simulink model "gm_uz_pmsm_model_6LUT_pd"  (R2023b)
settings: Solver=FixedStepAuto  StartTime=0.0  StopTime=0.05  RelTol=1e-3
PreLoadFcn:
  | uz_pmsm_model_init_parameter
PostLoadFcn:
  | % Import the data from Excel for a lookup table
  | FluxMapData = readtable('C:\Users\Philipp\ultrazohm\ultrazohm_sw\ip_cores\uz_pmsm_model\FluxMapData_2023-05-26_13-07-57.csv');
  | % Row indices for lookup table
  | d_current_in_d_axis = FluxMapData(8:27,1:end);
  | % Column indices for lookup table
  | q_current_in_d_axis = FluxMapData(29:48,1:end);
  | % Output values for lookup table
  | d_Flux_d_axis = FluxMapData(50:69,1:end);
undefined symbols (not defined in the file or in its folder): ad1, ad2, ad3, ad4, ad5, ad6, aq1, aq2, aq3, aq4, aq5, aq6, d_current_d_Flux, d_current_q_Flux, entkopplung_dynamic, entkopplung_linear, entkopplung_static, Fid1_Giq1, Fid2_Giq2, Flux_d, Flux_q, friction_coefficient, inertia, Ki_Bo_d, Ki_Bo_q, Kp_Bo_d, Kp_Bo_q, L_d, L_q, Ldq, parameter_nachfuerung, polepair, praediktion_entkopplung_nonlinear, psi_pm, q_current_d_Flux, q_current_q_Flux, R_1, simulate_mechanical, simulate_nonlinear_modell, simulate_open_loop, static_friction_torque, tau_sum, ts_regler
libraries: hdlmdlgenlib x21, slpidlib x2
(part 3 of 3)

== system gm_uz_pmsm_model_6LUT_pd/uz_pmsm_model/Product142 ==
  In1 : Inport
  In2 : Inport  Port=2
  Product142 : Product  Inputs=**  OutDataTypeStr=single  SampleTime=1e-08
  Product142_pd1 : Delay  DelayLength=6
  Out1 : Outport
  wires:
  In1/1 -> Product142/1
  In2/1 -> Product142/2
  Product142/1 -> Product142_pd1/1
  Product142_pd1/1 -> Out1/1

== system gm_uz_pmsm_model_6LUT_pd/uz_pmsm_model/Product15 ==
  In1 : Inport
  In2 : Inport  Port=2
  Product15 : Product  Inputs=**  OutDataTypeStr=single  SampleTime=1e-08
  Product15_pd1 : Delay  DelayLength=6
  Out1 : Outport
  wires:
  In1/1 -> Product15/1
  In2/1 -> Product15/2
  Product15/1 -> Product15_pd1/1
  Product15_pd1/1 -> Out1/1

== system gm_uz_pmsm_model_6LUT_pd/uz_pmsm_model/Product151 ==
  In1 : Inport
  In2 : Inport  Port=2
  Product151 : Product  Inputs=**  OutDataTypeStr=single  SampleTime=1e-08
  Product151_pd1 : Delay  DelayLength=6
  Out1 : Outport
  wires:
  In1/1 -> Product151/1
  In2/1 -> Product151/2
  Product151/1 -> Product151_pd1/1
  Product151_pd1/1 -> Out1/1

== system gm_uz_pmsm_model_6LUT_pd/uz_pmsm_model/Product16 ==
  In1 : Inport
  In2 : Inport  Port=2
  Product16 : Product  Inputs=**  OutDataTypeStr=single  SampleTime=1e-08
  Product16_pd1 : Delay  DelayLength=6
  Out1 : Outport
  wires:
  In1/1 -> Product16/1
  In2/1 -> Product16/2
  Product16/1 -> Product16_pd1/1
  Product16_pd1/1 -> Out1/1

== system gm_uz_pmsm_model_6LUT_pd/uz_pmsm_model/Product17 ==
  In1 : Inport
  In2 : Inport  Port=2
  Product17 : Product  Inputs=**  OutDataTypeStr=single  SampleTime=1e-08
  Product17_pd1 : Delay  DelayLength=6
  Out1 : Outport
  wires:
  In1/1 -> Product17/1
  In2/1 -> Product17/2
  Product17/1 -> Product17_pd1/1
  Product17_pd1/1 -> Out1/1

== system gm_uz_pmsm_model_6LUT_pd/uz_pmsm_model/Product18 ==
  In1 : Inport
  In2 : Inport  Port=2
  Product18 : Product  Inputs=**  OutDataTypeStr=single  SampleTime=1e-08
  Product18_pd1 : Delay  DelayLength=6
  Out1 : Outport
  wires:
  In1/1 -> Product18/1
  In2/1 -> Product18/2
  Product18/1 -> Product18_pd1/1
  Product18_pd1/1 -> Out1/1

== system gm_uz_pmsm_model_6LUT_pd/uz_pmsm_model/Product19 ==
  In1 : Inport
  In2 : Inport  Port=2
  Product19 : Product  Inputs=**  OutDataTypeStr=single  SampleTime=1e-08
  Product19_pd1 : Delay  DelayLength=6
  Out1 : Outport
  wires:
  In1/1 -> Product19/1
  In2/1 -> Product19/2
  Product19/1 -> Product19_pd1/1
  Product19_pd1/1 -> Out1/1

== system gm_uz_pmsm_model_6LUT_pd/uz_pmsm_model/Product2 ==
  In1 : Inport
  In2 : Inport  Port=2
  Product2 : Product  Inputs=**  OutDataTypeStr=single  SampleTime=1e-08
  Product2_pd1 : Delay  DelayLength=6
  Out1 : Outport
  wires:
  In1/1 -> Product2/1
  In2/1 -> Product2/2
  Product2/1 -> Product2_pd1/1
  Product2_pd1/1 -> Out1/1

== system gm_uz_pmsm_model_6LUT_pd/uz_pmsm_model/Product20 ==
  In1 : Inport
  In2 : Inport  Port=2
  Product20 : Product  Inputs=**  OutDataTypeStr=single  SampleTime=1e-08
  Product20_pd1 : Delay  DelayLength=6
  Out1 : Outport
  wires:
  In1/1 -> Product20/1
  In2/1 -> Product20/2
  Product20/1 -> Product20_pd1/1
  Product20_pd1/1 -> Out1/1

== system gm_uz_pmsm_model_6LUT_pd/uz_pmsm_model/Product201 ==
  In1 : Inport
  In2 : Inport  Port=2
  Product201 : Product  Inputs=**  OutDataTypeStr=single  SampleTime=1e-08
  Product201_pd1 : Delay  DelayLength=6
  Out1 : Outport
  wires:
  In1/1 -> Product201/1
  In2/1 -> Product201/2
  Product201/1 -> Product201_pd1/1
  Product201_pd1/1 -> Out1/1

== system gm_uz_pmsm_model_6LUT_pd/uz_pmsm_model/Product202 ==
  In1 : Inport
  In2 : Inport  Port=2
  Product202 : Product  Inputs=**  OutDataTypeStr=single  SampleTime=1e-08
  Product202_pd1 : Delay  DelayLength=6
  Out1 : Outport
  wires:
  In1/1 -> Product202/1
  In2/1 -> Product202/2
  Product202/1 -> Product202_pd1/1
  Product202_pd1/1 -> Out1/1

== system gm_uz_pmsm_model_6LUT_pd/uz_pmsm_model/Product203 ==
  In1 : Inport
  In2 : Inport  Port=2
  Product203 : Product  Inputs=**  OutDataTypeStr=single  SampleTime=1e-08
  Product203_pd1 : Delay  DelayLength=6
  Out1 : Outport
  wires:
  In1/1 -> Product203/1
  In2/1 -> Product203/2
  Product203/1 -> Product203_pd1/1
  Product203_pd1/1 -> Out1/1

== system gm_uz_pmsm_model_6LUT_pd/uz_pmsm_model/Product204 ==
  In1 : Inport
  In2 : Inport  Port=2
  Product204 : Product  Inputs=**  OutDataTypeStr=single  SampleTime=1e-08
  Product204_pd1 : Delay  DelayLength=6
  Out1 : Outport
  wires:
  In1/1 -> Product204/1
  In2/1 -> Product204/2
  Product204/1 -> Product204_pd1/1
  Product204_pd1/1 -> Out1/1

== system gm_uz_pmsm_model_6LUT_pd/uz_pmsm_model/Product205 ==
  In1 : Inport
  In2 : Inport  Port=2
  Product205 : Product  Inputs=**  OutDataTypeStr=single  SampleTime=1e-08
  Product205_pd1 : Delay  DelayLength=6
  Out1 : Outport
  wires:
  In1/1 -> Product205/1
  In2/1 -> Product205/2
  Product205/1 -> Product205_pd1/1
  Product205_pd1/1 -> Out1/1

== system gm_uz_pmsm_model_6LUT_pd/uz_pmsm_model/Product206 ==
  In1 : Inport
  In2 : Inport  Port=2
  Product206 : Product  Inputs=**  OutDataTypeStr=single  SampleTime=1e-08
  Product206_pd1 : Delay  DelayLength=6
  Out1 : Outport
  wires:
  In1/1 -> Product206/1
  In2/1 -> Product206/2
  Product206/1 -> Product206_pd1/1
  Product206_pd1/1 -> Out1/1

== system gm_uz_pmsm_model_6LUT_pd/uz_pmsm_model/Product207 ==
  In1 : Inport
  In2 : Inport  Port=2
  Product207 : Product  Inputs=**  OutDataTypeStr=single  SampleTime=1e-08
  Product207_pd1 : Delay  DelayLength=6
  Out1 : Outport
  wires:
  In1/1 -> Product207/1
  In2/1 -> Product207/2
  Product207/1 -> Product207_pd1/1
  Product207_pd1/1 -> Out1/1

== system gm_uz_pmsm_model_6LUT_pd/uz_pmsm_model/Product21 ==
  In1 : Inport
  In2 : Inport  Port=2
  Product21 : Product  Inputs=**  OutDataTypeStr=single  SampleTime=1e-08
  Product21_pd1 : Delay  DelayLength=6
  Out1 : Outport
  wires:
  In1/1 -> Product21/1
  In2/1 -> Product21/2
  Product21/1 -> Product21_pd1/1
  Product21_pd1/1 -> Out1/1

== system gm_uz_pmsm_model_6LUT_pd/uz_pmsm_model/Product22 ==
  In1 : Inport
  In2 : Inport  Port=2
  Product22 : Product  Inputs=**  OutDataTypeStr=single  SampleTime=1e-08
  Product22_pd1 : Delay  DelayLength=6
  Out1 : Outport
  wires:
  In1/1 -> Product22/1
  In2/1 -> Product22/2
  Product22/1 -> Product22_pd1/1
  Product22_pd1/1 -> Out1/1

== system gm_uz_pmsm_model_6LUT_pd/uz_pmsm_model/Product23 ==
  In1 : Inport
  In2 : Inport  Port=2
  Product23 : Product  Inputs=**  OutDataTypeStr=single  SampleTime=1e-08
  Product23_pd1 : Delay  DelayLength=6
  Out1 : Outport
  wires:
  In1/1 -> Product23/1
  In2/1 -> Product23/2
  Product23/1 -> Product23_pd1/1
  Product23_pd1/1 -> Out1/1

== system gm_uz_pmsm_model_6LUT_pd/uz_pmsm_model/Product24 ==
  In1 : Inport
  In2 : Inport  Port=2
  Product24 : Product  Inputs=**  OutDataTypeStr=single  SampleTime=1e-08
  Product24_pd1 : Delay  DelayLength=6
  Out1 : Outport
  wires:
  In1/1 -> Product24/1
  In2/1 -> Product24/2
  Product24/1 -> Product24_pd1/1
  Product24_pd1/1 -> Out1/1

== system gm_uz_pmsm_model_6LUT_pd/uz_pmsm_model/Product25 ==
  In1 : Inport
  In2 : Inport  Port=2
  Product25 : Product  Inputs=**  OutDataTypeStr=single  SampleTime=1e-08
  Product25_pd1 : Delay  DelayLength=6
  Out1 : Outport
  wires:
  In1/1 -> Product25/1
  In2/1 -> Product25/2
  Product25/1 -> Product25_pd1/1
  Product25_pd1/1 -> Out1/1

== system gm_uz_pmsm_model_6LUT_pd/uz_pmsm_model/Product3 ==
  In1 : Inport
  In2 : Inport  Port=2
  Product3 : Product  Inputs=**  OutDataTypeStr=single  SampleTime=1e-08
  Product3_pd1 : Delay  DelayLength=6
  Out1 : Outport
  wires:
  In1/1 -> Product3/1
  In2/1 -> Product3/2
  Product3/1 -> Product3_pd1/1
  Product3_pd1/1 -> Out1/1

== system gm_uz_pmsm_model_6LUT_pd/uz_pmsm_model/Product31 ==
  In1 : Inport
  In2 : Inport  Port=2
  Product31 : Product  Inputs=**  OutDataTypeStr=single  SampleTime=1e-08
  Product31_pd1 : Delay  DelayLength=6
  Out1 : Outport
  wires:
  In1/1 -> Product31/1
  In2/1 -> Product31/2
  Product31/1 -> Product31_pd1/1
  Product31_pd1/1 -> Out1/1

== system gm_uz_pmsm_model_6LUT_pd/uz_pmsm_model/Product32 ==
  In1 : Inport
  In2 : Inport  Port=2
  Product32 : Product  Inputs=**  OutDataTypeStr=single  SampleTime=1e-08
  Product32_pd1 : Delay  DelayLength=6
  Out1 : Outport
  wires:
  In1/1 -> Product32/1
  In2/1 -> Product32/2
  Product32/1 -> Product32_pd1/1
  Product32_pd1/1 -> Out1/1

== system gm_uz_pmsm_model_6LUT_pd/uz_pmsm_model/Product33 ==
  In1 : Inport
  In2 : Inport  Port=2
  Product33 : Product  Inputs=**  OutDataTypeStr=single  SampleTime=1e-08
  Product33_pd1 : Delay  DelayLength=6
  Out1 : Outport
  wires:
  In1/1 -> Product33/1
  In2/1 -> Product33/2
  Product33/1 -> Product33_pd1/1
  Product33_pd1/1 -> Out1/1

== system gm_uz_pmsm_model_6LUT_pd/uz_pmsm_model/Product34 ==
  In1 : Inport
  In2 : Inport  Port=2
  Product34 : Product  Inputs=**  OutDataTypeStr=single  SampleTime=1e-08
  Product34_pd1 : Delay  DelayLength=6
  Out1 : Outport
  wires:
  In1/1 -> Product34/1
  In2/1 -> Product34/2
  Product34/1 -> Product34_pd1/1
  Product34_pd1/1 -> Out1/1

== system gm_uz_pmsm_model_6LUT_pd/uz_pmsm_model/Product35 ==
  In1 : Inport
  In2 : Inport  Port=2
  Product35 : Product  Inputs=**  OutDataTypeStr=single  SampleTime=1e-08
  Product35_pd1 : Delay  DelayLength=6
  Out1 : Outport
  wires:
  In1/1 -> Product35/1
  In2/1 -> Product35/2
  Product35/1 -> Product35_pd1/1
  Product35_pd1/1 -> Out1/1

== system gm_uz_pmsm_model_6LUT_pd/uz_pmsm_model/Product4 ==
  In1 : Inport
  In2 : Inport  Port=2
  Product4 : Product  Inputs=**  OutDataTypeStr=single  SampleTime=1e-08
  Product4_pd1 : Delay  DelayLength=6
  Out1 : Outport
  wires:
  In1/1 -> Product4/1
  In2/1 -> Product4/2
  Product4/1 -> Product4_pd1/1
  Product4_pd1/1 -> Out1/1

== system gm_uz_pmsm_model_6LUT_pd/uz_pmsm_model/Product41 ==
  In1 : Inport
  In2 : Inport  Port=2
  Product41 : Product  Inputs=**  OutDataTypeStr=single  SampleTime=1e-08
  Product41_pd1 : Delay  DelayLength=6
  Out1 : Outport
  wires:
  In1/1 -> Product41/1
  In2/1 -> Product41/2
  Product41/1 -> Product41_pd1/1
  Product41_pd1/1 -> Out1/1

== system gm_uz_pmsm_model_6LUT_pd/uz_pmsm_model/Product42 ==
  In1 : Inport
  In2 : Inport  Port=2
  Product42 : Product  Inputs=**  OutDataTypeStr=single  SampleTime=1e-08
  Product42_pd1 : Delay  DelayLength=6
  Out1 : Outport
  wires:
  In1/1 -> Product42/1
  In2/1 -> Product42/2
  Product42/1 -> Product42_pd1/1
  Product42_pd1/1 -> Out1/1

== system gm_uz_pmsm_model_6LUT_pd/uz_pmsm_model/Product43 ==
  In1 : Inport
  In2 : Inport  Port=2
  Product43 : Product  Inputs=**  OutDataTypeStr=single  SampleTime=1e-08
  Product43_pd1 : Delay  DelayLength=6
  Out1 : Outport
  wires:
  In1/1 -> Product43/1
  In2/1 -> Product43/2
  Product43/1 -> Product43_pd1/1
  Product43_pd1/1 -> Out1/1

== system gm_uz_pmsm_model_6LUT_pd/uz_pmsm_model/Product5 ==
  In1 : Inport
  In2 : Inport  Port=2
  Product5 : Product  Inputs=**  OutDataTypeStr=single  SampleTime=1e-08
  Product5_pd1 : Delay  DelayLength=6
  Out1 : Outport
  wires:
  In1/1 -> Product5/1
  In2/1 -> Product5/2
  Product5/1 -> Product5_pd1/1
  Product5_pd1/1 -> Out1/1

== system gm_uz_pmsm_model_6LUT_pd/uz_pmsm_model/Product51 ==
  In1 : Inport
  In2 : Inport  Port=2
  Product51 : Product  Inputs=**  OutDataTypeStr=single  SampleTime=1e-08
  Product51_pd1 : Delay  DelayLength=6
  Out1 : Outport
  wires:
  In1/1 -> Product51/1
  In2/1 -> Product51/2
  Product51/1 -> Product51_pd1/1
  Product51_pd1/1 -> Out1/1

== system gm_uz_pmsm_model_6LUT_pd/uz_pmsm_model/Product52 ==
  In1 : Inport
  In2 : Inport  Port=2
  Product52 : Product  Inputs=**  OutDataTypeStr=single  SampleTime=1e-08
  Product52_pd1 : Delay  DelayLength=6
  Out1 : Outport
  wires:
  In1/1 -> Product52/1
  In2/1 -> Product52/2
  Product52/1 -> Product52_pd1/1
  Product52_pd1/1 -> Out1/1

== system gm_uz_pmsm_model_6LUT_pd/uz_pmsm_model/Product6 ==
  In1 : Inport
  In2 : Inport  Port=2
  Product6 : Product  Inputs=**  OutDataTypeStr=single  SampleTime=1e-08
  Product6_pd1 : Delay  DelayLength=6
  Out1 : Outport
  wires:
  In1/1 -> Product6/1
  In2/1 -> Product6/2
  Product6/1 -> Product6_pd1/1
  Product6_pd1/1 -> Out1/1

== system gm_uz_pmsm_model_6LUT_pd/uz_pmsm_model/Product61 ==
  In1 : Inport
  In2 : Inport  Port=2
  Product61 : Product  Inputs=**  OutDataTypeStr=single  SampleTime=1e-08
  Product61_pd1 : Delay  DelayLength=6
  Out1 : Outport
  wires:
  In1/1 -> Product61/1
  In2/1 -> Product61/2
  Product61/1 -> Product61_pd1/1
  Product61_pd1/1 -> Out1/1

== system gm_uz_pmsm_model_6LUT_pd/uz_pmsm_model/Product7 ==
  In1 : Inport
  In2 : Inport  Port=2
  Product7 : Product  Inputs=**  OutDataTypeStr=single  SampleTime=1e-08
  Product7_pd1 : Delay  DelayLength=6
  Out1 : Outport
  wires:
  In1/1 -> Product7/1
  In2/1 -> Product7/2
  Product7/1 -> Product7_pd1/1
  Product7_pd1/1 -> Out1/1

== system gm_uz_pmsm_model_6LUT_pd/uz_pmsm_model/Product71 ==
  In1 : Inport
  In2 : Inport  Port=2
  Product71 : Product  Inputs=**  OutDataTypeStr=single  SampleTime=1e-08
  Product71_pd1 : Delay  DelayLength=6
  Out1 : Outport
  wires:
  In1/1 -> Product71/1
  In2/1 -> Product71/2
  Product71/1 -> Product71_pd1/1
  Product71_pd1/1 -> Out1/1

== system gm_uz_pmsm_model_6LUT_pd/uz_pmsm_model/Product8 ==
  In1 : Inport
  In2 : Inport  Port=2
  Product8 : Product  Inputs=**  OutDataTypeStr=single  SampleTime=1e-08
  Product8_pd1 : Delay  DelayLength=6
  Out1 : Outport
  wires:
  In1/1 -> Product8/1
  In2/1 -> Product8/2
  Product8/1 -> Product8_pd1/1
  Product8_pd1/1 -> Out1/1

== system gm_uz_pmsm_model_6LUT_pd/uz_pmsm_model/Product9 ==
  In1 : Inport
  In2 : Inport  Port=2
  Product9 : Product  Inputs=**  OutDataTypeStr=single  SampleTime=1e-08
  Product9_pd1 : Delay  DelayLength=6
  Out1 : Outport
  wires:
  In1/1 -> Product9/1
  In2/1 -> Product9/2
  Product9/1 -> Product9_pd1/1
  Product9_pd1/1 -> Out1/1

== system gm_uz_pmsm_model_6LUT_pd/uz_pmsm_model/Product91 ==
  In1 : Inport
  In2 : Inport  Port=2
  Product91 : Product  Inputs=**  OutDataTypeStr=single  SampleTime=1e-08
  Product91_pd1 : Delay  DelayLength=6
  Out1 : Outport
  wires:
  In1/1 -> Product91/1
  In2/1 -> Product91/2
  Product91/1 -> Product91_pd1/1
  Product91_pd1/1 -> Out1/1

== system gm_uz_pmsm_model_6LUT_pd/uz_pmsm_model/Product92 ==
  In1 : Inport
  In2 : Inport  Port=2
  Product92 : Product  Inputs=**  OutDataTypeStr=single  SampleTime=1e-08
  Product92_pd1 : Delay  DelayLength=6
  Out1 : Outport
  wires:
  In1/1 -> Product92/1
  In2/1 -> Product92/2
  Product92/1 -> Product92_pd1/1
  Product92_pd1/1 -> Out1/1

== system gm_uz_pmsm_model_6LUT_pd/uz_pmsm_model/Reciprocal1_recip ==
  In1 : Inport
  Reciprocal1_recip : Math  Operator=reciprocal  SampleTime=1e-08
  Reciprocal1_recip_pd1 : Delay  DelayLength=16
  Out1 : Outport
  wires:
  In1/1 -> Reciprocal1_recip/1
  Reciprocal1_recip/1 -> Reciprocal1_recip_pd1/1
  Reciprocal1_recip_pd1/1 -> Out1/1

== system gm_uz_pmsm_model_6LUT_pd/uz_pmsm_model/Reciprocal1_recip1 ==
  In1 : Inport
  Reciprocal1_recip1 : Math  Operator=reciprocal  SampleTime=1e-08
  Reciprocal1_recip1_pd1 : Delay  DelayLength=16
  Out1 : Outport
  wires:
  In1/1 -> Reciprocal1_recip1/1
  Reciprocal1_recip1/1 -> Reciprocal1_recip1_pd1/1
  Reciprocal1_recip1_pd1/1 -> Out1/1

== system gm_uz_pmsm_model_6LUT_pd/uz_pmsm_model/Reciprocal_recip ==
  In1 : Inport
  Reciprocal_recip : Math  Operator=reciprocal  SampleTime=1e-08
  Reciprocal_recip_pd1 : Delay  DelayLength=16
  Out1 : Outport
  wires:
  In1/1 -> Reciprocal_recip/1
  Reciprocal_recip/1 -> Reciprocal_recip_pd1/1
  Reciprocal_recip_pd1/1 -> Out1/1

== system gm_uz_pmsm_model_6LUT_pd/uz_pmsm_model/Reciprocal_recip1 ==
  In1 : Inport
  Reciprocal_recip1 : Math  Operator=reciprocal  SampleTime=1e-08
  Reciprocal_recip1_pd1 : Delay  DelayLength=16
  Out1 : Outport
  wires:
  In1/1 -> Reciprocal_recip1/1
  Reciprocal_recip1/1 -> Reciprocal_recip1_pd1/1
  Reciprocal_recip1_pd1/1 -> Out1/1

== system gm_uz_pmsm_model_6LUT_pd/uz_pmsm_model/Sign1 ==
  In1 : Inport
  Sign1 : Signum  SampleTime=1e-08
  Out1 : Outport
  wires:
  In1/1 -> Sign1/1
  Sign1/1 -> Out1/1

== system gm_uz_pmsm_model_6LUT_pd/uz_pmsm_model/Sum ==
  In1 : Inport
  In2 : Inport  Port=2
  Sum : Sum  OutDataTypeStr=single  SampleTime=1e-08
  Sum_pd1 : Delay  DelayLength=6
  Out1 : Outport
  wires:
  In1/1 -> Sum/1
  In2/1 -> Sum/2
  Sum/1 -> Sum_pd1/1
  Sum_pd1/1 -> Out1/1

== system gm_uz_pmsm_model_6LUT_pd/uz_pmsm_model/Sum1 ==
  In1 : Inport
  In2 : Inport  Port=2
  Sum1 : Sum  Inputs=+-  OutDataTypeStr=single  SampleTime=1e-08
  Sum1_pd1 : Delay  DelayLength=6
  Out1 : Outport
  wires:
  In1/1 -> Sum1/1
  In2/1 -> Sum1/2
  Sum1/1 -> Sum1_pd1/1
  Sum1_pd1/1 -> Out1/1

== system gm_uz_pmsm_model_6LUT_pd/uz_pmsm_model/Sum10 ==
  In1 : Inport
  In2 : Inport  Port=2
  Sum10 : Sum  Inputs=+-  OutDataTypeStr=single  SampleTime=1e-08
  Sum10_pd1 : Delay  DelayLength=6
  Out1 : Outport
  wires:
  In1/1 -> Sum10/1
  In2/1 -> Sum10/2
  Sum10/1 -> Sum10_pd1/1
  Sum10_pd1/1 -> Out1/1

== system gm_uz_pmsm_model_6LUT_pd/uz_pmsm_model/Sum101 ==
  In1 : Inport
  In2 : Inport  Port=2
  Sum101 : Sum  Inputs=+-  OutDataTypeStr=single  SampleTime=1e-08
  Sum101_pd1 : Delay  DelayLength=6
  Out1 : Outport
  wires:
  In1/1 -> Sum101/1
  In2/1 -> Sum101/2
  Sum101/1 -> Sum101_pd1/1
  Sum101_pd1/1 -> Out1/1

== system gm_uz_pmsm_model_6LUT_pd/uz_pmsm_model/Sum11 ==
  In1 : Inport
  In2 : Inport  Port=2
  Sum11 : Sum  Inputs=+-  OutDataTypeStr=single  SampleTime=1e-08
  Sum11_pd1 : Delay  DelayLength=6
  Out1 : Outport
  wires:
  In1/1 -> Sum11/1
  In2/1 -> Sum11/2
  Sum11/1 -> Sum11_pd1/1
  Sum11_pd1/1 -> Out1/1

== system gm_uz_pmsm_model_6LUT_pd/uz_pmsm_model/Sum12 ==
  In1 : Inport
  In2 : Inport  Port=2
  Sum12 : Sum  OutDataTypeStr=single  SampleTime=1e-08
  Sum12_pd1 : Delay  DelayLength=6
  Out1 : Outport
  wires:
  In1/1 -> Sum12/1
  In2/1 -> Sum12/2
  Sum12/1 -> Sum12_pd1/1
  Sum12_pd1/1 -> Out1/1

== system gm_uz_pmsm_model_6LUT_pd/uz_pmsm_model/Sum13 ==
  In1 : Inport
  In2 : Inport  Port=2
  Sum13 : Sum  OutDataTypeStr=single  SampleTime=1e-08
  Sum13_pd1 : Delay  DelayLength=6
  Out1 : Outport
  wires:
  In1/1 -> Sum13/1
  In2/1 -> Sum13/2
  Sum13/1 -> Sum13_pd1/1
  Sum13_pd1/1 -> Out1/1

== system gm_uz_pmsm_model_6LUT_pd/uz_pmsm_model/Sum14 ==
  In1 : Inport
  In2 : Inport  Port=2
  Sum14 : Sum  Inputs=+-  OutDataTypeStr=single  SampleTime=1e-08
  Sum14_pd1 : Delay  DelayLength=6
  Out1 : Outport
  wires:
  In1/1 -> Sum14/1
  In2/1 -> Sum14/2
  Sum14/1 -> Sum14_pd1/1
  Sum14_pd1/1 -> Out1/1

== system gm_uz_pmsm_model_6LUT_pd/uz_pmsm_model/Sum2 ==
  In1 : Inport
  In2 : Inport  Port=2
  Sum2 : Sum  Inputs=+-  OutDataTypeStr=single  SampleTime=1e-08
  Sum2_pd1 : Delay  DelayLength=6
  Out1 : Outport
  wires:
  In1/1 -> Sum2/1
  In2/1 -> Sum2/2
  Sum2/1 -> Sum2_pd1/1
  Sum2_pd1/1 -> Out1/1

== system gm_uz_pmsm_model_6LUT_pd/uz_pmsm_model/Sum21 ==
  In1 : Inport
  In2 : Inport  Port=2
  Sum21 : Sum  Inputs=+-  OutDataTypeStr=single  SampleTime=1e-08
  Sum21_pd1 : Delay  DelayLength=6
  Out1 : Outport
  wires:
  In1/1 -> Sum21/1
  In2/1 -> Sum21/2
  Sum21/1 -> Sum21_pd1/1
  Sum21_pd1/1 -> Out1/1

== system gm_uz_pmsm_model_6LUT_pd/uz_pmsm_model/Sum22 ==
  In1 : Inport
  In2 : Inport  Port=2
  Sum22 : Sum  Inputs=+-  OutDataTypeStr=single  SampleTime=1e-08
  Sum22_pd1 : Delay  DelayLength=6
  Out1 : Outport
  wires:
  In1/1 -> Sum22/1
  In2/1 -> Sum22/2
  Sum22/1 -> Sum22_pd1/1
  Sum22_pd1/1 -> Out1/1

== system gm_uz_pmsm_model_6LUT_pd/uz_pmsm_model/Sum23 ==
  In1 : Inport
  In2 : Inport  Port=2
  Sum23 : Sum  Inputs=+-  OutDataTypeStr=single  SampleTime=1e-08
  Sum23_pd1 : Delay  DelayLength=6
  Out1 : Outport
  wires:
  In1/1 -> Sum23/1
  In2/1 -> Sum23/2
  Sum23/1 -> Sum23_pd1/1
  Sum23_pd1/1 -> Out1/1

== system gm_uz_pmsm_model_6LUT_pd/uz_pmsm_model/Sum3 ==
  In1 : Inport
  In2 : Inport  Port=2
  Sum3 : Sum  Inputs=+-  OutDataTypeStr=single  SampleTime=1e-08
  Sum3_pd1 : Delay  DelayLength=6
  Out1 : Outport
  wires:
  In1/1 -> Sum3/1
  In2/1 -> Sum3/2
  Sum3/1 -> Sum3_pd1/1
  Sum3_pd1/1 -> Out1/1

== system gm_uz_pmsm_model_6LUT_pd/uz_pmsm_model/Sum31 ==
  In1 : Inport
  In2 : Inport  Port=2
  Sum31 : Sum  Inputs=+-  OutDataTypeStr=single  SampleTime=1e-08
  Sum31_pd1 : Delay  DelayLength=6
  Out1 : Outport
  wires:
  In1/1 -> Sum31/1
  In2/1 -> Sum31/2
  Sum31/1 -> Sum31_pd1/1
  Sum31_pd1/1 -> Out1/1

== system gm_uz_pmsm_model_6LUT_pd/uz_pmsm_model/Sum32 ==
  In1 : Inport
  In2 : Inport  Port=2
  Sum32 : Sum  OutDataTypeStr=single  SampleTime=1e-08
  Sum32_pd1 : Delay  DelayLength=6
  Out1 : Outport
  wires:
  In1/1 -> Sum32/1
  In2/1 -> Sum32/2
  Sum32/1 -> Sum32_pd1/1
  Sum32_pd1/1 -> Out1/1

== system gm_uz_pmsm_model_6LUT_pd/uz_pmsm_model/Sum33 ==
  In1 : Inport
  In2 : Inport  Port=2
  Sum33 : Sum  Inputs=+-  OutDataTypeStr=single  SampleTime=1e-08
  Sum33_pd1 : Delay  DelayLength=6
  Out1 : Outport
  wires:
  In1/1 -> Sum33/1
  In2/1 -> Sum33/2
  Sum33/1 -> Sum33_pd1/1
  Sum33_pd1/1 -> Out1/1

== system gm_uz_pmsm_model_6LUT_pd/uz_pmsm_model/Sum3_stage2 ==
  In1 : Inport
  In2 : Inport  Port=2
  Sum3_stage2 : Sum  OutDataTypeStr=single  SampleTime=1e-08
  Sum3_stage2_pd1 : Delay  DelayLength=6
  Out1 : Outport
  wires:
  In1/1 -> Sum3_stage2/1
  In2/1 -> Sum3_stage2/2
  Sum3_stage2/1 -> Sum3_stage2_pd1/1
  Sum3_stage2_pd1/1 -> Out1/1

== system gm_uz_pmsm_model_6LUT_pd/uz_pmsm_model/Sum3_stage21 ==
  In1 : Inport
  In2 : Inport  Port=2
  Sum3_stage21 : Sum  Inputs=+-  OutDataTypeStr=single  SampleTime=1e-08
  Sum3_stage21_pd1 : Delay  DelayLength=6
  Out1 : Outport
  wires:
  In1/1 -> Sum3_stage21/1
  In2/1 -> Sum3_stage21/2
  Sum3_stage21/1 -> Sum3_stage21_pd1/1
  Sum3_stage21_pd1/1 -> Out1/1

== system gm_uz_pmsm_model_6LUT_pd/uz_pmsm_model/Sum3_stage3 ==
  In1 : Inport
  In2 : Inport  Port=2
  Sum3_stage3 : Sum  Inputs=+-  OutDataTypeStr=single  SampleTime=1e-08
  Sum3_stage3_pd1 : Delay  DelayLength=6
  Out1 : Outport
  wires:
  In1/1 -> Sum3_stage3/1
  In2/1 -> Sum3_stage3/2
  Sum3_stage3/1 -> Sum3_stage3_pd1/1
  Sum3_stage3_pd1/1 -> Out1/1

== system gm_uz_pmsm_model_6LUT_pd/uz_pmsm_model/Sum3_stage31 ==
  In1 : Inport
  In2 : Inport  Port=2
  Sum3_stage31 : Sum  Inputs=+-  OutDataTypeStr=single  SampleTime=1e-08
  Sum3_stage31_pd1 : Delay  DelayLength=6
  Out1 : Outport
  wires:
  In1/1 -> Sum3_stage31/1
  In2/1 -> Sum3_stage31/2
  Sum3_stage31/1 -> Sum3_stage31_pd1/1
  Sum3_stage31_pd1/1 -> Out1/1

== system gm_uz_pmsm_model_6LUT_pd/uz_pmsm_model/Sum3_stage4 ==
  In1 : Inport
  In2 : Inport  Port=2
  Sum3_stage4 : Sum  OutDataTypeStr=single  SampleTime=1e-08
  Sum3_stage4_pd1 : Delay  DelayLength=6
  Out1 : Outport
  wires:
  In1/1 -> Sum3_stage4/1
  In2/1 -> Sum3_stage4/2
  Sum3_stage4/1 -> Sum3_stage4_pd1/1
  Sum3_stage4_pd1/1 -> Out1/1

== system gm_uz_pmsm_model_6LUT_pd/uz_pmsm_model/Sum4 ==
  In1 : Inport
  In2 : Inport  Port=2
  Sum4 : Sum  Inputs=+-  OutDataTypeStr=single  SampleTime=1e-08
  Sum4_pd1 : Delay  DelayLength=6
  Out1 : Outport
  wires:
  In1/1 -> Sum4/1
  In2/1 -> Sum4/2
  Sum4/1 -> Sum4_pd1/1
  Sum4_pd1/1 -> Out1/1

== system gm_uz_pmsm_model_6LUT_pd/uz_pmsm_model/Sum41 ==
  In1 : Inport
  In2 : Inport  Port=2
  Sum41 : Sum  OutDataTypeStr=single  SampleTime=1e-08
  Sum41_pd1 : Delay  DelayLength=6
  Out1 : Outport
  wires:
  In1/1 -> Sum41/1
  In2/1 -> Sum41/2
  Sum41/1 -> Sum41_pd1/1
  Sum41_pd1/1 -> Out1/1

== system gm_uz_pmsm_model_6LUT_pd/uz_pmsm_model/Sum42 ==
  In1 : Inport
  In2 : Inport  Port=2
  Sum42 : Sum  OutDataTypeStr=single  SampleTime=1e-08
  Sum42_pd1 : Delay  DelayLength=6
  Out1 : Outport
  wires:
  In1/1 -> Sum42/1
  In2/1 -> Sum42/2
  Sum42/1 -> Sum42_pd1/1
  Sum42_pd1/1 -> Out1/1

== system gm_uz_pmsm_model_6LUT_pd/uz_pmsm_model/Sum4_stage2 ==
  In1 : Inport
  In2 : Inport  Port=2
  Sum4_stage2 : Sum  Inputs=+-  OutDataTypeStr=single  SampleTime=1e-08
  Sum4_stage2_pd1 : Delay  DelayLength=6
  Out1 : Outport
  wires:
  In1/1 -> Sum4_stage2/1
  In2/1 -> Sum4_stage2/2
  Sum4_stage2/1 -> Sum4_stage2_pd1/1
  Sum4_stage2_pd1/1 -> Out1/1

== system gm_uz_pmsm_model_6LUT_pd/uz_pmsm_model/Sum4_stage3 ==
  In1 : Inport
  In2 : Inport  Port=2
  Sum4_stage3 : Sum  Inputs=+-  OutDataTypeStr=single  SampleTime=1e-08
  Sum4_stage3_pd1 : Delay  DelayLength=6
  Out1 : Outport
  wires:
  In1/1 -> Sum4_stage3/1
  In2/1 -> Sum4_stage3/2
  Sum4_stage3/1 -> Sum4_stage3_pd1/1
  Sum4_stage3_pd1/1 -> Out1/1

== system gm_uz_pmsm_model_6LUT_pd/uz_pmsm_model/Sum4_stage4 ==
  In1 : Inport
  In2 : Inport  Port=2
  Sum4_stage4 : Sum  Inputs=+-  OutDataTypeStr=single  SampleTime=1e-08
  Sum4_stage4_pd1 : Delay  DelayLength=6
  Out1 : Outport
  wires:
  In1/1 -> Sum4_stage4/1
  In2/1 -> Sum4_stage4/2
  Sum4_stage4/1 -> Sum4_stage4_pd1/1
  Sum4_stage4_pd1/1 -> Out1/1

== system gm_uz_pmsm_model_6LUT_pd/uz_pmsm_model/Sum5 ==
  In1 : Inport
  In2 : Inport  Port=2
  Sum5 : Sum  Inputs=+-  OutDataTypeStr=single  SampleTime=1e-08
  Sum5_pd1 : Delay  DelayLength=6
  Out1 : Outport
  wires:
  In1/1 -> Sum5/1
  In2/1 -> Sum5/2
  Sum5/1 -> Sum5_pd1/1
  Sum5_pd1/1 -> Out1/1

== system gm_uz_pmsm_model_6LUT_pd/uz_pmsm_model/Sum51 ==
  In1 : Inport
  In2 : Inport  Port=2
  Sum51 : Sum  OutDataTypeStr=single  SampleTime=1e-08
  Sum51_pd1 : Delay  DelayLength=6
  Out1 : Outport
  wires:
  In1/1 -> Sum51/1
  In2/1 -> Sum51/2
  Sum51/1 -> Sum51_pd1/1
  Sum51_pd1/1 -> Out1/1

== system gm_uz_pmsm_model_6LUT_pd/uz_pmsm_model/Sum52 ==
  In1 : Inport
  In2 : Inport  Port=2
  Sum52 : Sum  OutDataTypeStr=single  SampleTime=1e-08
  Sum52_pd1 : Delay  DelayLength=6
  Out1 : Outport
  wires:
  In1/1 -> Sum52/1
  In2/1 -> Sum52/2
  Sum52/1 -> Sum52_pd1/1
  Sum52_pd1/1 -> Out1/1

== system gm_uz_pmsm_model_6LUT_pd/uz_pmsm_model/Sum53 ==
  In1 : Inport
  In2 : Inport  Port=2
  Sum53 : Sum  OutDataTypeStr=single  SampleTime=1e-08
  Sum53_pd1 : Delay  DelayLength=6
  Out1 : Outport
  wires:
  In1/1 -> Sum53/1
  In2/1 -> Sum53/2
  Sum53/1 -> Sum53_pd1/1
  Sum53_pd1/1 -> Out1/1

== system gm_uz_pmsm_model_6LUT_pd/uz_pmsm_model/Sum6 ==
  In1 : Inport
  In2 : Inport  Port=2
  Sum6 : Sum  Inputs=+-  OutDataTypeStr=single  SampleTime=1e-08
  Sum6_pd1 : Delay  DelayLength=6
  Out1 : Outport
  wires:
  In1/1 -> Sum6/1
  In2/1 -> Sum6/2
  Sum6/1 -> Sum6_pd1/1
  Sum6_pd1/1 -> Out1/1

== system gm_uz_pmsm_model_6LUT_pd/uz_pmsm_model/Sum7 ==
  In1 : Inport
  In2 : Inport  Port=2
  Sum7 : Sum  Inputs=+-  OutDataTypeStr=single  SampleTime=1e-08
  Sum7_pd1 : Delay  DelayLength=6
  Out1 : Outport
  wires:
  In1/1 -> Sum7/1
  In2/1 -> Sum7/2
  Sum7/1 -> Sum7_pd1/1
  Sum7_pd1/1 -> Out1/1

== system gm_uz_pmsm_model_6LUT_pd/uz_pmsm_model/Sum71 ==
  In1 : Inport
  In2 : Inport  Port=2
  Sum71 : Sum  Inputs=+-  OutDataTypeStr=single  SampleTime=1e-08
  Sum71_pd1 : Delay  DelayLength=6
  Out1 : Outport
  wires:
  In1/1 -> Sum71/1
  In2/1 -> Sum71/2
  Sum71/1 -> Sum71_pd1/1
  Sum71_pd1/1 -> Out1/1

== system gm_uz_pmsm_model_6LUT_pd/uz_pmsm_model/Sum8 ==
  In1 : Inport
  In2 : Inport  Port=2
  Sum8 : Sum  Inputs=+-  OutDataTypeStr=single  SampleTime=1e-08
  Sum8_pd1 : Delay  DelayLength=6
  Out1 : Outport
  wires:
  In1/1 -> Sum8/1
  In2/1 -> Sum8/2
  Sum8/1 -> Sum8_pd1/1
  Sum8_pd1/1 -> Out1/1

== system gm_uz_pmsm_model_6LUT_pd/uz_pmsm_model/Tanh ==
  In1 : Inport
  Tanh : Trigonometry  Operator=tanh  SampleTime=1e-08
  Tanh_pd1 : Delay  DelayLength=25
  Out1 : Outport
  wires:
  In1/1 -> Tanh/1
  Tanh/1 -> Tanh_pd1/1
  Tanh_pd1/1 -> Out1/1

== system gm_uz_pmsm_model_6LUT_pd/uz_pmsm_model/Tanh1 ==
  In1 : Inport
  Tanh1 : Trigonometry  Operator=cosh  SampleTime=1e-08
  Tanh1_pd1 : Delay  DelayLength=17
  Out1 : Outport
  wires:
  In1/1 -> Tanh1/1
  Tanh1/1 -> Tanh1_pd1/1
  Tanh1_pd1/1 -> Out1/1

== system gm_uz_pmsm_model_6LUT_pd/uz_pmsm_model/Tanh11 ==
  In1 : Inport
  Tanh11 : Trigonometry  Operator=tanh  SampleTime=1e-08
  Tanh11_pd1 : Delay  DelayLength=25
  Out1 : Outport
  wires:
  In1/1 -> Tanh11/1
  Tanh11/1 -> Tanh11_pd1/1
  Tanh11_pd1/1 -> Out1/1

== system gm_uz_pmsm_model_6LUT_pd/uz_pmsm_model/Tanh12 ==
  In1 : Inport
  Tanh12 : Trigonometry  Operator=tanh  SampleTime=1e-08
  Tanh12_pd1 : Delay  DelayLength=25
  Out1 : Outport
  wires:
  In1/1 -> Tanh12/1
  Tanh12/1 -> Tanh12_pd1/1
  Tanh12_pd1/1 -> Out1/1

== system gm_uz_pmsm_model_6LUT_pd/uz_pmsm_model/Tanh13 ==
  In1 : Inport
  Tanh13 : Trigonometry  Operator=cosh  SampleTime=1e-08
  Tanh13_pd1 : Delay  DelayLength=17
  Out1 : Outport
  wires:
  In1/1 -> Tanh13/1
  Tanh13/1 -> Tanh13_pd1/1
  Tanh13_pd1/1 -> Out1/1

== system gm_uz_pmsm_model_6LUT_pd/uz_pmsm_model/Tanh2 ==
  In1 : Inport
  Tanh2 : Trigonometry  Operator=cosh  SampleTime=1e-08
  Tanh2_pd1 : Delay  DelayLength=17
  Out1 : Outport
  wires:
  In1/1 -> Tanh2/1
  Tanh2/1 -> Tanh2_pd1/1
  Tanh2_pd1/1 -> Out1/1

== system gm_uz_pmsm_model_6LUT_pd/uz_pmsm_model/Tanh21 ==
  In1 : Inport
  Tanh21 : Trigonometry  Operator=cosh  SampleTime=1e-08
  Tanh21_pd1 : Delay  DelayLength=17
  Out1 : Outport
  wires:
  In1/1 -> Tanh21/1
  Tanh21/1 -> Tanh21_pd1/1
  Tanh21_pd1/1 -> Out1/1

== system gm_uz_pmsm_model_6LUT_pd/uz_pmsm_model/Tanh3 ==
  In1 : Inport
  Tanh3 : Trigonometry  Operator=cosh  SampleTime=1e-08
  Tanh3_pd1 : Delay  DelayLength=17
  Out1 : Outport
  wires:
  In1/1 -> Tanh3/1
  Tanh3/1 -> Tanh3_pd1/1
  Tanh3_pd1/1 -> Out1/1

== system gm_uz_pmsm_model_6LUT_pd/uz_pmsm_model/Tanh31 ==
  In1 : Inport
  Tanh31 : Trigonometry  Operator=cosh  SampleTime=1e-08
  Tanh31_pd1 : Delay  DelayLength=17
  Out1 : Outport
  wires:
  In1/1 -> Tanh31/1
  Tanh31/1 -> Tanh31_pd1/1
  Tanh31_pd1/1 -> Out1/1

== system gm_uz_pmsm_model_6LUT_pd/uz_pmsm_model/Tanh4 ==
  In1 : Inport
  Tanh4 : Trigonometry  Operator=cosh  SampleTime=1e-08
  Tanh4_pd1 : Delay  DelayLength=17
  Out1 : Outport
  wires:
  In1/1 -> Tanh4/1
  Tanh4/1 -> Tanh4_pd1/1
  Tanh4_pd1/1 -> Out1/1

== system gm_uz_pmsm_model_6LUT_pd/uz_pmsm_model/Tanh41 ==
  In1 : Inport
  Tanh41 : Trigonometry  Operator=cosh  SampleTime=1e-08
  Tanh41_pd1 : Delay  DelayLength=17
  Out1 : Outport
  wires:
  In1/1 -> Tanh41/1
  Tanh41/1 -> Tanh41_pd1/1
  Tanh41_pd1/1 -> Out1/1

== system gm_uz_pmsm_model_6LUT_pd/uz_pmsm_model/Tanh5 ==
  In1 : Inport
  Tanh5 : Trigonometry  Operator=tanh  SampleTime=1e-08
  Tanh5_pd1 : Delay  DelayLength=25
  Out1 : Outport
  wires:
  In1/1 -> Tanh5/1
  Tanh5/1 -> Tanh5_pd1/1
  Tanh5_pd1/1 -> Out1/1

== system gm_uz_pmsm_model_6LUT_pd/Current_Controller/Entkopplungen/Lineare_Entkopplung ==
  i_d : Inport
  i_q : Inport  Port=2
  omega_m : Inport  Port=3
  Constant1 : Constant  Value=psi_pm  SampleTime=-1
  Gain : Gain  Gain=L_q
  Gain1 : Gain  Gain=L_d
  Gain2 : Gain  Gain=polepair
  Product : Product
  Product1 : Product
  Sum6 : Sum  Inputs=|++
  u_d : Outport
  u_q : Outport  Port=2
  wires:
  Gain/1 -> Product/1
  Gain2/1 -> Product/2, Product1/2
  Gain1/1 -> Sum6/1
  Product1/1 -> u_q/1
  i_q/1 -> Gain/1
  Constant1/1 -> Sum6/2
  i_d/1 -> Gain1/1
  Product/1 -> u_d/1
  Sum6/1 -> Product1/1
  omega_m/1 -> Gain2/1

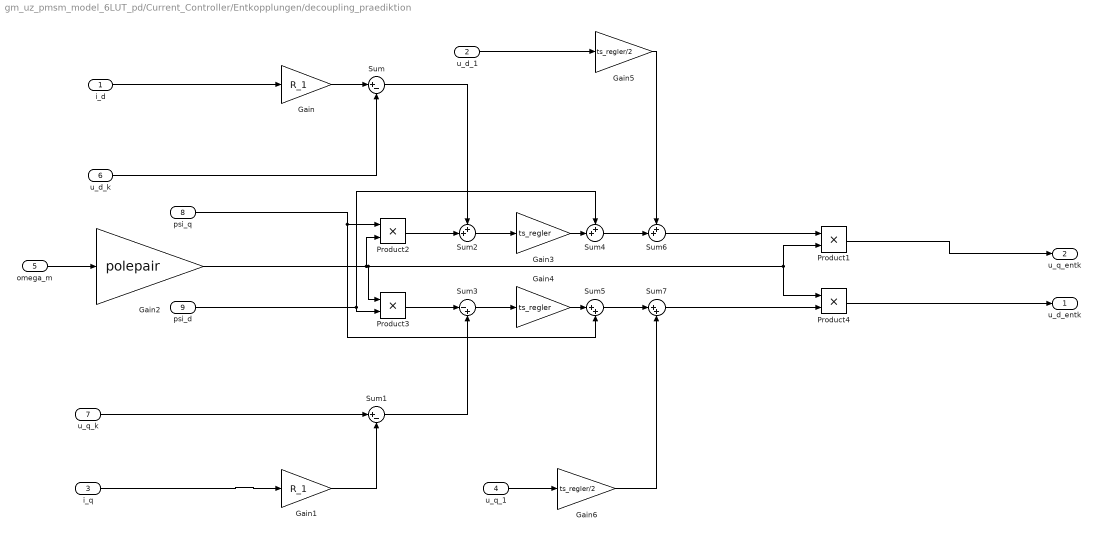
== system gm_uz_pmsm_model_6LUT_pd/Current_Controller/Entkopplungen/decoupling_praediktion ==
  i_d : Inport
  u_d_1 : Inport  Port=2
  i_q : Inport  Port=3
  u_q_1 : Inport  Port=4
  omega_m : Inport  Port=5
  u_d_k : Inport  Port=6
  u_q_k : Inport  Port=7
  psi_q : Inport  Port=8
  psi_d : Inport  Port=9
  Gain : Gain  Gain=R_1
  Gain1 : Gain  Gain=R_1
  Gain2 : Gain  Gain=polepair
  Gain3 : Gain  Gain=ts_regler
  Gain4 : Gain  Gain=ts_regler
  Gain5 : Gain  Gain=ts_regler/2
  Gain6 : Gain  Gain=ts_regler/2
  Product{1..4} (4 alike) : Product
  Sum : Sum  Inputs=|+-
  Sum1 : Sum  Inputs=|+-
  Sum2 : Sum  Inputs=++|
  Sum3 : Sum  Inputs=|-+
  Sum4 : Sum  Inputs=++|
  Sum5 : Sum  Inputs=|++
  Sum6 : Sum  Inputs=++|
  Sum7 : Sum  Inputs=|++
  u_d_entk : Outport
  u_q_entk : Outport  Port=2
  wires:
  Product4/1 -> u_d_entk/1
  Product1/1 -> u_q_entk/1
  i_q/1 -> Gain1/1
  i_d/1 -> Gain/1
  omega_m/1 -> Gain2/1
  Sum7/1 -> Product4/2
  Sum6/1 -> Product1/1
  Gain6/1 -> Sum7/2
  Sum5/1 -> Sum7/1
  Gain5/1 -> Sum6/1
  u_q_1/1 -> Gain6/1
  Sum4/1 -> Sum6/2
  u_d_1/1 -> Gain5/1
  Gain4/1 -> Sum5/1
  Gain3/1 -> Sum4/2
  Sum2/1 -> Gain3/1
  Sum3/1 -> Gain4/1
  Sum1/1 -> Sum3/2
  Sum/1 -> Sum2/1
  Product2/1 -> Sum2/2
  Product3/1 -> Sum3/1
  Gain1/1 -> Sum1/2
  u_q_k/1 -> Sum1/1
  Gain/1 -> Sum/1
  u_d_k/1 -> Sum/2
  Gain2/1 -> Product2/2, Product3/1, Product4/1, Product1/2
  psi_d/1 -> Sum4/1, Product3/2
  psi_q/1 -> Product2/1, Sum5/2

== system gm_uz_pmsm_model_6LUT_pd/Current_Controller/Entkopplungen/dynamic_nonlinear_entkopplung1 ==
  i_d : Inport
  i_q : Inport  Port=2
  psi_d : Inport  Port=3
  psi_q : Inport  Port=4
  Ldq_LUT : Inport  Port=5
  Lqd_LUT : Inport  Port=6
  omega_m : Inport  Port=7
  Gain2 : Gain  Gain=polepair
  Product{,1..3} (4 alike) : Product
  Sum1 : Sum  Inputs=++|
  Sum6 : Sum  Inputs=++|
  u_d : Outport
  u_q : Outport  Port=2
  wires:
  Product2/1 -> Sum1/1
  Product3/1 -> Sum6/1
  Lqd_LUT/1 -> Product3/2
  i_q/1 -> Product3/1
  Sum1/1 -> u_d/1
  Product/1 -> Sum1/2
  Product1/1 -> Sum6/2
  Sum6/1 -> u_q/1
  Ldq_LUT/1 -> Product2/2
  i_d/1 -> Product2/1
  omega_m/1 -> Gain2/1
  psi_d/1 -> Product1/1  "psi_d_LUT"
  Gain2/1 -> Product/2, Product1/2
  psi_q/1 -> Product/1  "psi_q_LUT"

== system gm_uz_pmsm_model_6LUT_pd/Current_Controller/Entkopplungen/static_nonlinear_entkopplung ==
  psi_d : Inport
  psi_q : Inport  Port=2
  omega_m : Inport  Port=3
  Gain2 : Gain  Gain=polepair
  Product : Product
  Product1 : Product
  Scope : Scope  NumInputPorts=2
  u_d : Outport
  u_q : Outport  Port=2
  wires:
  omega_m/1 -> Gain2/1
  psi_d/1 -> Product1/1  "psi_d_LUT"
  Product/1 -> u_d/1, Scope/2
  Product1/1 -> u_q/1, Scope/1
  Gain2/1 -> Product/2, Product1/2
  psi_q/1 -> Product/1  "psi_q_LUT"
